simulink model "Proj3_P3"  (Simulink 8.6)
settings: Solver=ode45  StartTime=0.0  StopTime=90  FixedStep=1e-4  MaxStep=1e-4  RelTol=1e-3
values from neighbouring files (symbols this model uses):
  A = 3904    [main.m]
  ControlQs = 1    [main.m]
  ControlVwind = -1    [main.m]
  fl_rd_rated = L_m*I_sd_rated + L_r*I_rd_rated    [main.m]
  fl_rq_rated = L_m*I_sq_rated + L_r*I_rq_rated    [main.m]
  fl_sd_rated = L_s*I_sd_rated + L_m*I_rd_rated    [main.m]
  fl_sq_rated = L_s*I_sq_rated + L_m*I_rq_rated    [main.m]
  GearRatio = w_mech_rated / w_mech_opt    [main.m]
  J_turb = 2.4*10^6    (= 2400000)    [main.m]
  K_opt = Cp_opt * 0.5 * rho * A * R^3/lambda_opt^3    (= -inf)    [main.m]
  kii = w_c_i*sqrt(R_r^2+(sigma*L_r*w_c_i)^2)/sqrt(1+(kpi_by_kii*w_c_i)^2)    [main.m]
  kpi = kpi_by_kii * kii    [main.m]
  L_m = X_m /w_syn    (= 0.00228122085098)    [main.m]
  L_r = L_lr+L_m    (= 0.00240589222307)    [main.m]
  L_s = L_ls+L_m    (= 0.00241384997023)    [main.m]
  lambda_opt = lam    (= 0.01)    [main.m]
  p = 6    [main.m]
  Q_s_rated = (V_sd_rated)^2/(w_syn*L_s)+(L_m/L_s)*V_sd_rated*I_rq_rated    [main.m]
  R = 70.5/2    (= 35.25)    [main.m]
  R_r = 1.5e-3    (= 0.0015)    [main.m]
  R_s = 2e-3    (= 0.002)    [main.m]
  rho = 1.2    [main.m]
  sigma = 1-L_m^2/(L_s*L_r)    (= 0.10391703115)    [main.m]
  V_ll_rated = 690    [main.m]
  V_sd_prime_rated = V_rd_rated + s*w_syn*sigma*L_r*I_rq_rated    [main.m]
  V_sd_rated = V_ll_rated    (= 690)    [main.m]
  V_sq_prime_rated = V_rq_rated - s*w_syn*sigma*L_r*I_rd_rated    [main.m]
  v_wind = [12; 9; 6]    [main.m]
  w_mech_opt = lambda_opt*v_wind(1)/R    [main.m]
  w_mech_rated = (1-s)*w_syn/(p/2)    (= 124.407069082)    [main.m]
  w_syn = 2*pi*f_rated    (= 376.991118431)    [main.m]
settings Model: Creator=Admin  LastModifiedBy=XP
settings OptimizationCC: ExpressionDepthLimit=128
settings DebuggingCC: FcnCallInpInsideContextMsg=UseLocalSettings  StateNameClashWarn=none

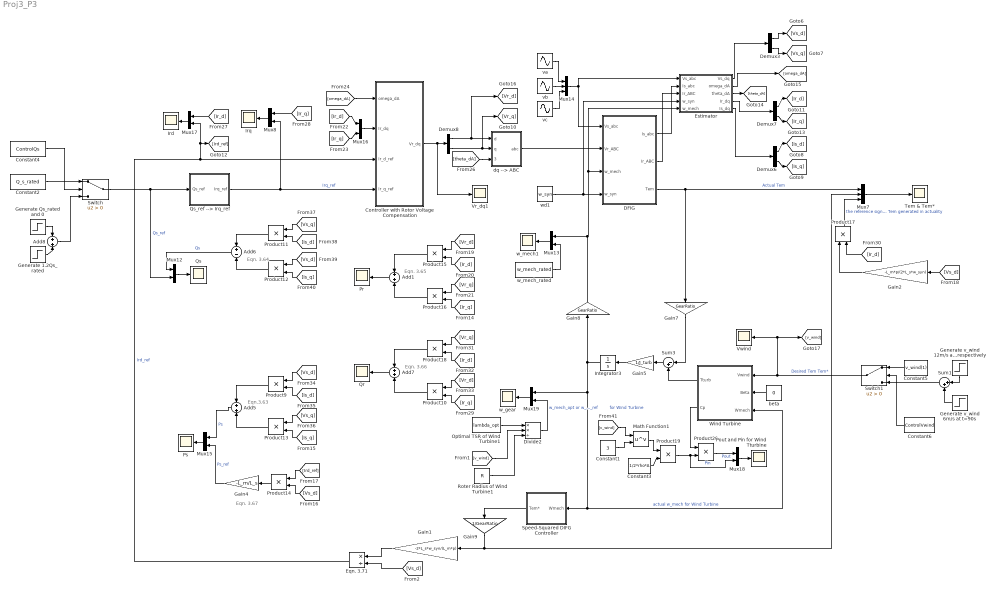
== system Proj3_P3 ==
  note: Eqn. 3.64
  note: Eqn. 3.66
  note: Eqn. 3.65
  note: Eqn.3.63
  note: Eqn. 3.67
  " Gain4" : Gain  Gain=-L_m/L_s
  " Gain5" : Gain  Gain=1/J_turb
  Add{1,5,7..8} (4 alike) : Sum
  Add6 : Sum  Inputs=+-
  Constant1 : Constant  Value=3
  Constant2 : Constant  Value=Q_s_rated
  Constant3 : Constant  Value=1/2*rho*A
  Constant4 : Constant  Value=ControlQs
  Constant5 : Constant  Value=v_wind(1)
  Constant6 : Constant  Value=ControlVwind
  Controller with Rotor Voltage Compensation : Subsystem
  DFIG : Subsystem
  Demux{3,6..8} (4 alike) : Demux  Outputs=2
  Divide2 : Product  Inputs=**/
  "Eqn. 3.71 " : Product  Inputs=*/
  Estimator : Subsystem
  Gain1 : Gain  Gain=-2*L_s*w_syn/(L_m*p)
  Gain2 : Gain  Gain=-L_m*p/(2*L_s*w_syn)
  Gain7 : Gain  Gain=GearRatio
  Gain8 : Gain  Gain=GearRatio
  Gain9 : Gain  Gain=1/GearRatio
  Generate Qs_rated and 0 : Step  Time=30  Before=Q_s_rated  After=0  SampleTime=0
  Generate 1.2Qs_rated : Step  Time=60  After=1.2*Q_s_rated  SampleTime=0
  Generate v_wind 12m/s and 9m/s at t=0s and t=60s respectively : Step  Time=30  Before=v_wind(1)  After=v_wind(2)  SampleTime=0
  Generate v_wind 6m/s at t=90s : Step  Time=60  After=v_wind(3)-v_wind(2)  SampleTime=0
  Integrator3 : Integrator  InitialCondition=w_mech_opt
  Ird : Scope
  Irq : Scope
  Math Function1 : Math  Operator=pow  SaturateOnIntegerOverflow=on
  Mux{8,12..13,15..19} (8 alike) : Mux  Inputs=2
  Mux14 : Mux  Inputs=3
  Mux7 : Mux  Inputs=3
  Optimal TSR of Wind Turbine1 : Constant  Value=lambda_opt
  Pout and Pin for Wind Tturbine : Scope
  Pr : Scope
  Product{9..20} (12 alike) : Product
  Ps : Scope
  Qr : Scope
  Qs : Scope
  Qs_ref --> Irq_ref : Subsystem
  Roter Radius of Wind Turbine1 : Constant  Value=R
  Speed-Squared DIFG Controller : Subsystem
  Sum1 : Sum  Inputs=|++
  Sum3 : Sum  Inputs=|-+
  Switch : Switch  Criteria=u2 > Threshold
  Switch1 : Switch  Criteria=u2 > Threshold
  Tem & Tem* : Scope
  Vr_dq1 : Scope
  Vwind : Scope
  Wind Turbine : Subsystem
  beta : Constant  Value=0
  dq --> ABC : Subsystem
  va : Sin  Amplitude=V_ll_rated*sqrt(2/3)  Frequency=2*pi*60  Phase=pi/2  SampleTime=0
  vb : Sin  Amplitude=V_ll_rated*sqrt(2/3)  Frequency=2*pi*60  Phase=pi/2-2*pi/3  SampleTime=0
  vc : Sin  Amplitude=V_ll_rated*sqrt(2/3)  Frequency=2*pi*60  Phase=pi/2+2*pi/3  SampleTime=0
  w_gear : Scope
  w_mech1 : Scope
  w_mech_rated : Constant  Value=w_mech_rated
  wd1 : Constant  Value=w_syn
  wires:
  dq --> ABC/1(abc) -> DFIG/2(Vr_ABC)
  vb/1 -> Mux14/2
  vc/1 -> Mux14/3
  va/1 -> Mux14/1
  Mux14/1 -> Estimator/1(Vs_abc), DFIG/1(Vs_abc)
  Demux8/1 -> dq --> ABC/1(d), [Vr_d]
  Demux8/2 -> [Vr_q], dq --> ABC/2(q)
  Controller with Rotor Voltage Compensation/1(Vr_dq) -> Vr_dq1/1, Demux8/1
  Mux17/1 -> Ird/1
  wd1/1 -> Estimator/4(w_syn), DFIG/4(w_syn)
  Estimator/1(Vs_dq) -> Demux3/1
  Mux7/1 -> Tem & Tem*/1
  "Eqn. 3.71 "/1 -> Controller with Rotor Voltage Compensation/3(Ir_d_ref), [Ird_ref], Mux17/2  "Ird_ref"
  Demux3/1 -> [Vs_d]
  Demux3/2 -> [Vs_q]
  Mux12/1 -> Qs/1
  DFIG/1(Is_abc) -> Estimator/2(Is_abc)
  DFIG/2(Ir_ABC) -> Estimator/3(Ir_ABC)
  Mux13/1 -> w_mech1/1
  w_mech_rated/1 -> Mux13/2
  Estimator/5(Is_dq) -> Demux6/1
  Demux6/1 -> [Is_d]
  Demux6/2 -> [Is_q]
  Add6/1 -> Mux12/1  "Qs"
  [Vs_q] -> Product11/1
  [Is_d] -> Product11/2
  [Vs_d] -> Product12/1
  [Is_q] -> Product12/2
  Product11/1 -> Add6/1
  Product12/1 -> Add6/2
  Switch/1 -> Mux12/2, Qs_ref --> Irq_ref/1(Qs_ref)  "Qs_ref"
  [Vs_d] -> Product9/1
  [Is_d] -> Product9/2
  [Vs_q] -> Product13/1
  [Is_q] -> Product13/2
  Product9/1 -> Add5/1
  Product13/1 -> Add5/2
  Add5/1 -> Mux15/1  "Ps"
  Estimator/2(omega_dA) -> [omega_dA]
  Gain8/1 -> Estimator/5(w_mech), DFIG/3(w_mech), Mux13/1
  [Vr_d] -> Product15/1
  [Ir_d] -> Product15/2
  [Vr_q] -> Product16/1
  [Ir_q] -> Product16/2
  Product15/1 -> Add1/1
  Product16/1 -> Add1/2
  Add1/1 -> Pr/1
  Estimator/4(Ir_dq) -> Demux7/1
  Demux7/1 -> [Ir_d]
  Demux7/2 -> [Ir_q]
  Estimator/3(theta_dA) -> [theta_dA]
  Mux16/1 -> Controller with Rotor Voltage Compensation/2(Ir_dq)
  [Ir_d] -> Mux16/1
  [Ir_q] -> Mux16/2
  [omega_dA] -> Controller with Rotor Voltage Compensation/1(omega_dA)
  [theta_dA] -> dq --> ABC/3(theta_dA)
  [Ir_d] -> Mux17/1
  Qs_ref --> Irq_ref/1(Irq_ref) -> Controller with Rotor Voltage Compensation/4(Ir_q_ref), Mux8/2  "Irq_ref"
  Mux8/1 -> Irq/1
  [Ir_q] -> Mux8/1
  [Vr_q] -> Product18/1
  [Ir_d] -> Product18/2
  [Vr_d] -> Product10/1
  [Ir_q] -> Product10/2
  Product18/1 -> Add7/1
  Product10/1 -> Add7/2
  Add7/1 -> Qr/1
  [Vs_d] -> Gain2/1
  [Ir_d] -> Product17/2
  Product17/1 -> Mux7/3  "the reference signal of Tem generated in actuality"
  Gain9/1 -> Gain1/1, Mux7/2  "Desired Tem Tem*"
  Gain2/1 -> Product17/1
  DFIG/3(Tem) -> Mux7/1, Gain7/1  "Actual Tem"
  Gain7/1 -> Sum3/1
  Sum3/1 -> " Gain5"/1
  " Gain5"/1 -> Integrator3/1
  Wind Turbine/1(Tturb) -> Sum3/2
  beta/1 -> Wind Turbine/2(Beta)
  [v_wind] -> Math Function1/1
  Constant1/1 -> Math Function1/2
  Constant3/1 -> Product19/2
  Math Function1/1 -> Product19/1
  Product19/1 -> Mux18/2, Product20/2  "Pin"
  Wind Turbine/2(Cp) -> Product20/1
  Product20/1 -> Mux18/1  "Pout"
  Mux18/1 -> Pout and Pin for Wind Tturbine/1
  Speed-Squared DIFG Controller/1(Tem*) -> Gain9/1
  Mux19/1 -> w_gear/1
  Divide2/1 -> Mux19/2  "w_mech_opt or w_mech_ref         for Wind Turbine"
  Integrator3/1 -> Gain8/1, Mux19/1, Speed-Squared DIFG Controller/1(Wmech), Wind Turbine/3(Wmech)  "actual w_mech for Wind Turbine"
  [v_wind] -> Divide2/2
  Optimal TSR of Wind Turbine1/1 -> Divide2/1
  Roter Radius of Wind Turbine1/1 -> Divide2/3
  Generate Qs_rated and 0/1 -> Add8/1
  Generate 1.2Qs_rated/1 -> Add8/2
  Constant2/1 -> Switch/1
  Add8/1 -> Switch/3
  Constant4/1 -> Switch/2
  Sum1/1 -> Switch1/3
  Generate v_wind 6m/s at t=90s/1 -> Sum1/2
  Generate v_wind 12m/s and 9m/s at t=0s and t=60s respectively/1 -> Sum1/1
  Constant5/1 -> Switch1/1
  [Vs_d] -> "Eqn. 3.71 "/2
  Gain1/1 -> "Eqn. 3.71 "/1
  Switch1/1 -> [v_wind], Vwind/1, Wind Turbine/1(Vwind)
  Constant6/1 -> Switch1/2
  [Vs_d] -> Product14/2
  [Ird_ref] -> Product14/1
  Product14/1 -> " Gain4"/1
  " Gain4"/1 -> Mux15/2  "Ps_ref"
  Mux15/1 -> Ps/1

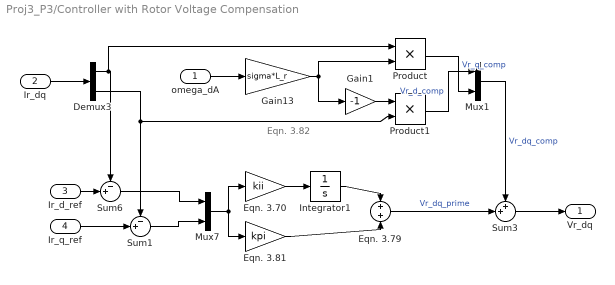
== system Proj3_P3/Controller with Rotor Voltage Compensation ==
  note: Eqn. 3.82
  omega_dA : Inport
  Ir_dq : Inport  Port=2
  Ir_d_ref : Inport  Port=3
  Ir_q_ref : Inport  Port=4
  "                       Eqn. 3.79" : Sum
  Demux3 : Demux  Outputs=2
  Eqn. 3.70 : Gain  Gain=kii
  Eqn. 3.81 : Gain  Gain=kpi
  Gain1 : Gain  Gain=-1
  Gain13 : Gain  Gain=sigma*L_r
  Integrator1 : Integrator  InitialCondition=[V_sd_prime_rated; V_sq_prime_rated]
  Mux1 : Mux  Inputs=2
  Mux7 : Mux  Inputs=2
  Product : Product
  Product1 : Product
  Sum1 : Sum  Inputs=-+|  SaturateOnIntegerOverflow=on  InputSameDT=on  OutDataTypeStr=Inherit: Same as first input
  Sum3 : Sum  Inputs=++|  SaturateOnIntegerOverflow=on  InputSameDT=on  OutDataTypeStr=Inherit: Same as first input
  Sum6 : Sum  Inputs=-+|  SaturateOnIntegerOverflow=on  InputSameDT=on  OutDataTypeStr=Inherit: Same as first input
  Vr_dq : Outport
  wires:
  Eqn. 3.70/1 -> Integrator1/1
  Integrator1/1 -> "                       Eqn. 3.79"/1
  Eqn. 3.81/1 -> "                       Eqn. 3.79"/2
  Mux7/1 -> Eqn. 3.81/1, Eqn. 3.70/1
  "                       Eqn. 3.79"/1 -> Sum3/2  "Vr_dq_prime"
  Demux3/2 -> Sum1/1, Product1/2
  Gain1/1 -> Product1/1
  Product1/1 -> Mux1/1  "Vr_d_comp"
  Gain13/1 -> Product/2, Gain1/1
  Product/1 -> Mux1/2  "Vr_q_comp"
  omega_dA/1 -> Gain13/1
  Ir_dq/1 -> Demux3/1
  Demux3/1 -> Sum6/1, Product/1
  Mux1/1 -> Sum3/1  "Vr_dq_comp"
  Sum3/1 -> Vr_dq/1
  Ir_d_ref/1 -> Sum6/2
  Ir_q_ref/1 -> Sum1/2
  Sum1/1 -> Mux7/2
  Sum6/1 -> Mux7/1

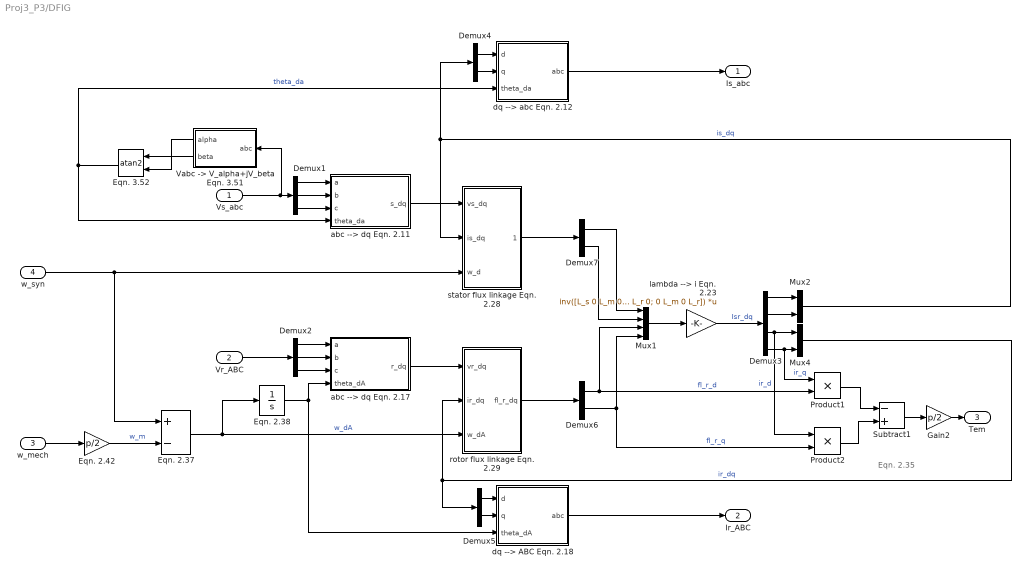
== system Proj3_P3/DFIG ==
  note: Eqn. 2.35
  Vs_abc : Inport
  Vr_ABC : Inport  Port=2
  w_mech : Inport  Port=3
  w_syn : Inport  Port=4
  Demux1 : Demux  Outputs=3
  Demux2 : Demux  Outputs=3
  Demux3 : Demux
  Demux{4..7} (4 alike) : Demux  Outputs=2
  Eqn. 2.37 : Sum  Inputs=+-
  Eqn. 2.38 : Integrator
  Eqn. 2.42 : Gain  Gain=p/2  SaturateOnIntegerOverflow=on  OutDataTypeStr=Inherit: Same as input  ParamDataTypeStr=Inherit: Same as input
  Eqn. 3.52 : Trigonometry  Operator=atan2
  Gain2 : Gain  Gain=p/2  SaturateOnIntegerOverflow=on  OutDataTypeStr=Inherit: Same as input  ParamDataTypeStr=Inherit: Same as input
  Mux1 : Mux
  Mux2 : Mux  Inputs=2
  Mux4 : Mux  Inputs=2
  Product1 : Product
  Product2 : Product
  Subtract1 : Sum  Inputs=-+
  "Vabc -> V_alpha+jV_beta Eqn. 3.51" : Subsystem
  abc --> dq Eqn. 2.11 : Subsystem
  abc --> dq Eqn. 2.17 : Subsystem
  dq --> ABC Eqn. 2.18 : Subsystem
  dq --> abc Eqn. 2.12 : Subsystem
  lambda --> i Eqn. 2.23 : Gain  Gain=inv([L_s 0 L_m 0; 0 L_s 0 L_m; L_m 0 L_r 0; 0 L_m 0 L_r])  Multiplication=Matrix(K*u)  SaturateOnIntegerOverflow=on  OutDataTypeStr=Inherit: Same as input  ParamDataTypeStr=Inherit: Same as input
  rotor flux linkage Eqn. 2.29 : Subsystem
  stator flux linkage Eqn. 2.28 : Subsystem
  Is_abc : Outport
  Ir_ABC : Outport  Port=2
  Tem : Outport  Port=3
  wires:
  Product2/1 -> Subtract1/2
  Vr_ABC/1 -> Demux2/1
  lambda --> i Eqn. 2.23/1 -> Demux3/1  "Isr_dq"
  Mux4/1 -> Demux5/1, rotor flux linkage Eqn. 2.29/2(ir_dq)  "ir_dq"
  Eqn. 2.37/1 -> rotor flux linkage Eqn. 2.29/3(w_dA), Eqn. 2.38/1  "w_dA"
  Demux4/1 -> dq --> abc Eqn. 2.12/1(d)
  Demux2/3 -> abc --> dq Eqn. 2.17/3(c)
  Demux2/1 -> abc --> dq Eqn. 2.17/1(a)
  Demux2/2 -> abc --> dq Eqn. 2.17/2(b)
  Eqn. 3.52/1 -> dq --> abc Eqn. 2.12/3(theta_da), abc --> dq Eqn. 2.11/4(theta_da)  "theta_da"
  Mux1/1 -> lambda --> i Eqn. 2.23/1
  Demux7/2 -> Mux1/2
  abc --> dq Eqn. 2.11/1(s_dq) -> stator flux linkage Eqn. 2.28/1(vs_dq)
  w_mech/1 -> Eqn. 2.42/1
  Demux4/2 -> dq --> abc Eqn. 2.12/2(q)
  Demux6/2 -> Mux1/4, Product2/2  "fl_r_q"
  Demux1/3 -> abc --> dq Eqn. 2.11/3(c)
  Eqn. 2.42/1 -> Eqn. 2.37/2  "w_m"
  Product1/1 -> Subtract1/1
  Eqn. 2.38/1 -> dq --> ABC Eqn. 2.18/3(theta_dA), abc --> dq Eqn. 2.17/4(theta_dA)
  Demux1/1 -> abc --> dq Eqn. 2.11/1(a)
  Demux5/1 -> dq --> ABC Eqn. 2.18/1(d)
  Demux5/2 -> dq --> ABC Eqn. 2.18/2(q)
  abc --> dq Eqn. 2.17/1(r_dq) -> rotor flux linkage Eqn. 2.29/1(vr_dq)
  rotor flux linkage Eqn. 2.29/1(fl_r_dq) -> Demux6/1
  Mux2/1 -> Demux4/1, stator flux linkage Eqn. 2.28/2(is_dq)  "is_dq"
  Demux6/1 -> Product1/2, Mux1/3  "fl_r_d"
  w_syn/1 -> stator flux linkage Eqn. 2.28/3(w_d), Eqn. 2.37/1
  dq --> abc Eqn. 2.12/1(abc) -> Is_abc/1
  Vs_abc/1 -> "Vabc -> V_alpha+jV_beta Eqn. 3.51"/1(abc), Demux1/1
  "Vabc -> V_alpha+jV_beta Eqn. 3.51"/2(beta) -> Eqn. 3.52/1
  dq --> ABC Eqn. 2.18/1(abc) -> Ir_ABC/1
  "Vabc -> V_alpha+jV_beta Eqn. 3.51"/1(alpha) -> Eqn. 3.52/2
  stator flux linkage Eqn. 2.28/1(fl_s_dq) -> Demux7/1
  Demux3/4 -> Product1/1, Mux4/2  "ir_q"
  Subtract1/1 -> Gain2/1
  Demux3/1 -> Mux2/1
  Demux3/3 -> Product2/1, Mux4/1  "ir_d"
  Demux3/2 -> Mux2/2
  Demux7/1 -> Mux1/1
  Gain2/1 -> Tem/1
  Demux1/2 -> abc --> dq Eqn. 2.11/2(b)

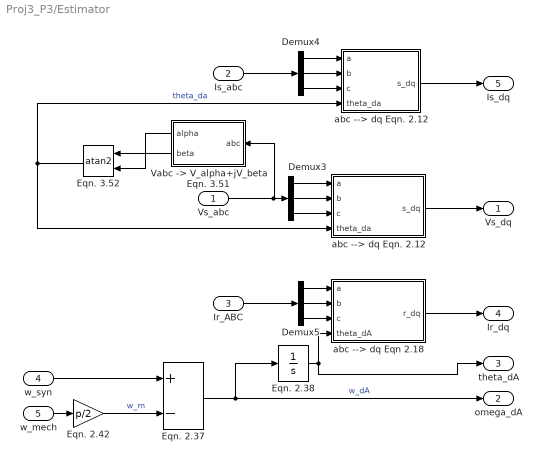
== system Proj3_P3/Estimator ==
  Vs_abc : Inport
  Is_abc : Inport  Port=2
  Ir_ABC : Inport  Port=3
  w_syn : Inport  Port=4
  w_mech : Inport  Port=5
  Demux3 : Demux  Outputs=3
  Demux4 : Demux  Outputs=3
  Demux5 : Demux  Outputs=3
  Eqn. 2.37 : Sum  Inputs=+-
  Eqn. 2.38 : Integrator
  Eqn. 2.42 : Gain  Gain=p/2  SaturateOnIntegerOverflow=on  OutDataTypeStr=Inherit: Same as input  ParamDataTypeStr=Inherit: Same as input
  Eqn. 3.52 : Trigonometry  Operator=atan2
  "Vabc -> V_alpha+jV_beta Eqn. 3.51" : Subsystem
  abc --> dq Eqn 2.18 : Subsystem
  abc --> dq Eqn. 2.12 : Subsystem
  "abc --> dq Eqn. 2.12 " : Subsystem
  Vs_dq : Outport
  omega_dA : Outport  Port=2
  theta_dA : Outport  Port=3
  Ir_dq : Outport  Port=4
  Is_dq : Outport  Port=5
  wires:
  Eqn. 3.52/1 -> "abc --> dq Eqn. 2.12 "/4(theta_da), abc --> dq Eqn. 2.12/4(theta_da)  "theta_da"
  "abc --> dq Eqn. 2.12 "/1(s_dq) -> Vs_dq/1
  Demux3/3 -> "abc --> dq Eqn. 2.12 "/3(c)
  Demux3/1 -> "abc --> dq Eqn. 2.12 "/1(a)
  Vs_abc/1 -> "Vabc -> V_alpha+jV_beta Eqn. 3.51"/1(abc), Demux3/1
  "Vabc -> V_alpha+jV_beta Eqn. 3.51"/2(beta) -> Eqn. 3.52/1
  "Vabc -> V_alpha+jV_beta Eqn. 3.51"/1(alpha) -> Eqn. 3.52/2
  Demux3/2 -> "abc --> dq Eqn. 2.12 "/2(b)
  Demux4/1 -> abc --> dq Eqn. 2.12/1(a)
  Demux4/2 -> abc --> dq Eqn. 2.12/2(b)
  Demux4/3 -> abc --> dq Eqn. 2.12/3(c)
  Is_abc/1 -> Demux4/1
  Demux5/1 -> abc --> dq Eqn 2.18/1(a)
  Demux5/2 -> abc --> dq Eqn 2.18/2(b)
  Demux5/3 -> abc --> dq Eqn 2.18/3(c)
  Ir_ABC/1 -> Demux5/1
  Eqn. 2.37/1 -> omega_dA/1, Eqn. 2.38/1  "w_dA"
  w_mech/1 -> Eqn. 2.42/1
  Eqn. 2.42/1 -> Eqn. 2.37/2  "w_m"
  w_syn/1 -> Eqn. 2.37/1
  Eqn. 2.38/1 -> theta_dA/1, abc --> dq Eqn 2.18/4(theta_dA)
  abc --> dq Eqn 2.18/1(r_dq) -> Ir_dq/1
  abc --> dq Eqn. 2.12/1(s_dq) -> Is_dq/1

== system Proj3_P3/Qs_ref --> Irq_ref ==
  note: Eqn. 3.72
  Qs_ref : Inport
  Constant1 : Constant  Value=V_sd_rated/(w_syn*L_m)
  Gain7 : Gain  Gain=L_s/(L_m*V_sd_rated)
  Sum2 : Sum  Inputs=|+-
  Irq_ref : Outport
  wires:
  Qs_ref/1 -> Gain7/1
  Constant1/1 -> Sum2/2
  Gain7/1 -> Sum2/1
  Sum2/1 -> Irq_ref/1  "Irq_ref"

== system Proj3_P3/Speed-Squared DIFG Controller ==
  Wmech : Inport
  "Tem*=Kopt * Wmech^2 Eqn. 4.91 " : Fcn  Expr=K_opt*u^2
  Tem* : Outport
  wires:
  "Tem*=Kopt * Wmech^2 Eqn. 4.91 "/1 -> Tem*/1
  Wmech/1 -> "Tem*=Kopt * Wmech^2 Eqn. 4.91 "/1

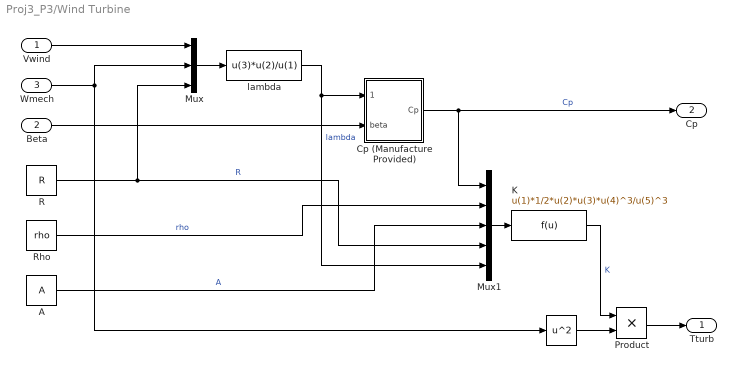
== system Proj3_P3/Wind Turbine ==
  Vwind : Inport
  Beta : Inport  Port=2
  Wmech : Inport  Port=3
  " " : Fcn  Expr=u^2
  A : Constant  Value=A
  Cp (Manufacture Provided) : Subsystem
  K : Fcn  Expr=u(1)*1/2*u(2)*u(3)*u(4)^3/u(5)^3
  Mux : Mux  Inputs=3
  Mux1 : Mux  Inputs=5
  Product : Product
  R : Constant  Value=R
  Rho : Constant  Value=rho
  lambda : Fcn  Expr=u(3)*u(2)/u(1)
  Tturb : Outport
  Cp : Outport  Port=2
  wires:
  lambda/1 -> Mux1/5, Cp (Manufacture Provided)/1(lambda)  "lambda"
  K/1 -> Product/1  "K"
  A/1 -> Mux1/3  "A"
  Mux1/1 -> K/1
  Mux/1 -> lambda/1
  Cp (Manufacture Provided)/1(Cp) -> Mux1/1, Cp/1  "Cp"
  " "/1 -> Product/2
  Product/1 -> Tturb/1
  Rho/1 -> Mux1/2  "rho"
  R/1 -> Mux/3, Mux1/4  "R"
  Vwind/1 -> Mux/1
  Wmech/1 -> Mux/2, " "/1
  Beta/1 -> Cp (Manufacture Provided)/2(beta)

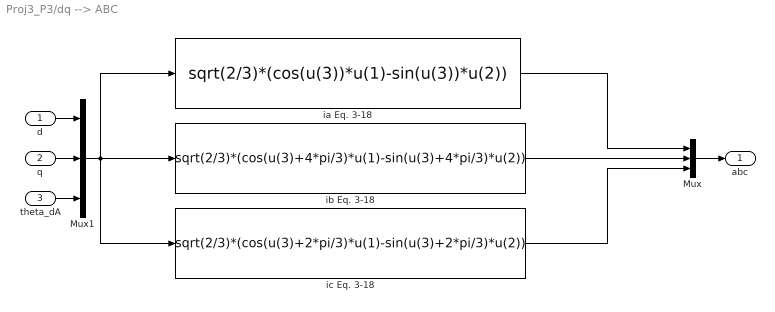
== system Proj3_P3/dq --> ABC ==
  d : Inport
  q : Inport  Port=2
  theta_dA : Inport  Port=3
  Mux : Mux  Inputs=3
  Mux1 : Mux  Inputs=3
  ia Eq. 3-18 : Fcn  Expr=sqrt(2/3)*(cos(u(3))*u(1)-sin(u(3))*u(2))
  ib Eq. 3-18 : Fcn  Expr=sqrt(2/3)*(cos(u(3)+4*pi/3)*u(1)-sin(u(3)+4*pi/3)*u(2))
  ic Eq. 3-18 : Fcn  Expr=sqrt(2/3)*(cos(u(3)+2*pi/3)*u(1)-sin(u(3)+2*pi/3)*u(2))
  abc : Outport
  wires:
  Mux/1 -> abc/1
  ia Eq. 3-18/1 -> Mux/1
  ic Eq. 3-18/1 -> Mux/3
  ib Eq. 3-18/1 -> Mux/2
  theta_dA/1 -> Mux1/3
  q/1 -> Mux1/2
  d/1 -> Mux1/1
  Mux1/1 -> ia Eq. 3-18/1, ib Eq. 3-18/1, ic Eq. 3-18/1

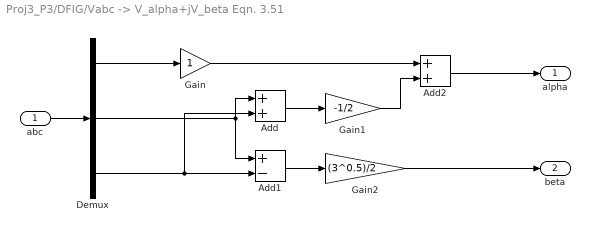
== system Proj3_P3/DFIG/Vabc -> V_alpha+jV_beta Eqn. 3.51 ==
  abc : Inport
  Add : Sum
  Add1 : Sum  Inputs=+-
  Add2 : Sum
  Demux : Demux  Outputs=3
  Gain : Gain
  Gain1 : Gain  Gain=-1/2
  Gain2 : Gain  Gain=(3^0.5)/2
  alpha : Outport
  beta : Outport  Port=2
  wires:
  Add/1 -> Gain1/1
  Add1/1 -> Gain2/1
  Demux/2 -> Add1/1, Add/1
  Demux/1 -> Gain/1
  Gain1/1 -> Add2/2
  Gain/1 -> Add2/1
  Add2/1 -> alpha/1
  Gain2/1 -> beta/1
  Demux/3 -> Add1/2, Add/2
  abc/1 -> Demux/1

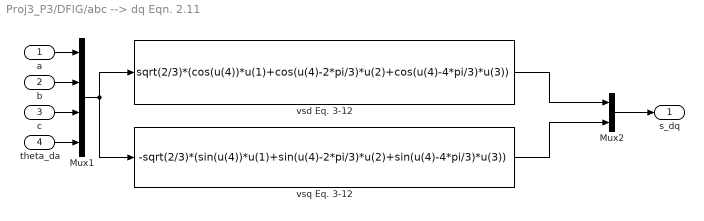
== system Proj3_P3/DFIG/abc --> dq Eqn. 2.11 ==
  a : Inport
  b : Inport  Port=2
  c : Inport  Port=3
  theta_da : Inport  Port=4
  Mux1 : Mux
  Mux2 : Mux  Inputs=2
  vsd Eq. 3-12 : Fcn  Expr=sqrt(2/3)*(cos(u(4))*u(1)+cos(u(4)-2*pi/3)*u(2)+cos(u(4)-4*pi/3)*u(3))
  vsq Eq. 3-12 : Fcn  Expr=-sqrt(2/3)*(sin(u(4))*u(1)+sin(u(4)-2*pi/3)*u(2)+sin(u(4)-4*pi/3)*u(3))
  s_dq : Outport
  wires:
  Mux1/1 -> vsd Eq. 3-12/1, vsq Eq. 3-12/1
  vsd Eq. 3-12/1 -> Mux2/1
  vsq Eq. 3-12/1 -> Mux2/2
  a/1 -> Mux1/1
  b/1 -> Mux1/2
  c/1 -> Mux1/3
  theta_da/1 -> Mux1/4
  Mux2/1 -> s_dq/1

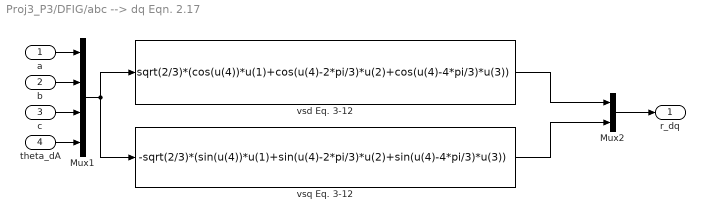
== system Proj3_P3/DFIG/abc --> dq Eqn. 2.17 ==
  a : Inport
  b : Inport  Port=2
  c : Inport  Port=3
  theta_dA : Inport  Port=4
  Mux1 : Mux
  Mux2 : Mux  Inputs=2
  vsd Eq. 3-12 : Fcn  Expr=sqrt(2/3)*(cos(u(4))*u(1)+cos(u(4)-2*pi/3)*u(2)+cos(u(4)-4*pi/3)*u(3))
  vsq Eq. 3-12 : Fcn  Expr=-sqrt(2/3)*(sin(u(4))*u(1)+sin(u(4)-2*pi/3)*u(2)+sin(u(4)-4*pi/3)*u(3))
  r_dq : Outport
  wires:
  Mux1/1 -> vsd Eq. 3-12/1, vsq Eq. 3-12/1
  vsd Eq. 3-12/1 -> Mux2/1
  vsq Eq. 3-12/1 -> Mux2/2
  a/1 -> Mux1/1
  b/1 -> Mux1/2
  c/1 -> Mux1/3
  theta_dA/1 -> Mux1/4
  Mux2/1 -> r_dq/1

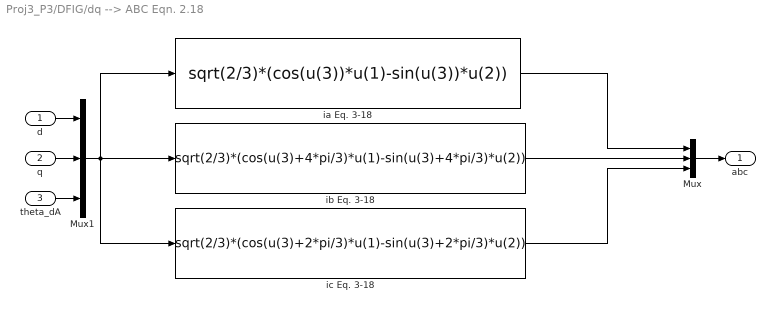
== system Proj3_P3/DFIG/dq --> ABC Eqn. 2.18 ==
  d : Inport
  q : Inport  Port=2
  theta_dA : Inport  Port=3
  Mux : Mux  Inputs=3
  Mux1 : Mux  Inputs=3
  ia Eq. 3-18 : Fcn  Expr=sqrt(2/3)*(cos(u(3))*u(1)-sin(u(3))*u(2))
  ib Eq. 3-18 : Fcn  Expr=sqrt(2/3)*(cos(u(3)+4*pi/3)*u(1)-sin(u(3)+4*pi/3)*u(2))
  ic Eq. 3-18 : Fcn  Expr=sqrt(2/3)*(cos(u(3)+2*pi/3)*u(1)-sin(u(3)+2*pi/3)*u(2))
  abc : Outport
  wires:
  Mux1/1 -> ic Eq. 3-18/1, ib Eq. 3-18/1, ia Eq. 3-18/1
  d/1 -> Mux1/1
  q/1 -> Mux1/2
  theta_dA/1 -> Mux1/3
  ib Eq. 3-18/1 -> Mux/2
  ic Eq. 3-18/1 -> Mux/3
  ia Eq. 3-18/1 -> Mux/1
  Mux/1 -> abc/1

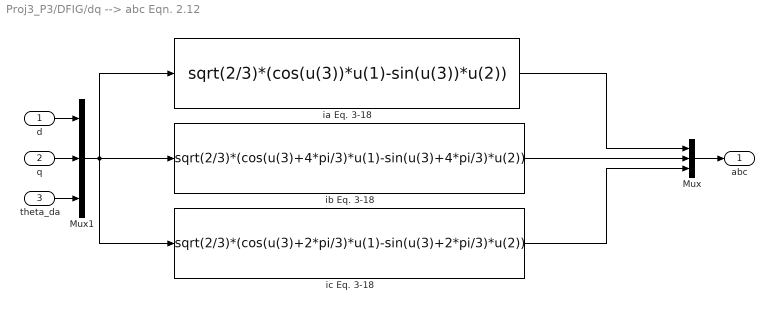
== system Proj3_P3/DFIG/dq --> abc Eqn. 2.12 ==
  d : Inport
  q : Inport  Port=2
  theta_da : Inport  Port=3
  Mux : Mux  Inputs=3
  Mux1 : Mux  Inputs=3
  ia Eq. 3-18 : Fcn  Expr=sqrt(2/3)*(cos(u(3))*u(1)-sin(u(3))*u(2))
  ib Eq. 3-18 : Fcn  Expr=sqrt(2/3)*(cos(u(3)+4*pi/3)*u(1)-sin(u(3)+4*pi/3)*u(2))
  ic Eq. 3-18 : Fcn  Expr=sqrt(2/3)*(cos(u(3)+2*pi/3)*u(1)-sin(u(3)+2*pi/3)*u(2))
  abc : Outport
  wires:
  Mux1/1 -> ic Eq. 3-18/1, ib Eq. 3-18/1, ia Eq. 3-18/1
  d/1 -> Mux1/1
  q/1 -> Mux1/2
  theta_da/1 -> Mux1/3
  ib Eq. 3-18/1 -> Mux/2
  ic Eq. 3-18/1 -> Mux/3
  ia Eq. 3-18/1 -> Mux/1
  Mux/1 -> abc/1

== system Proj3_P3/DFIG/rotor flux linkage Eqn. 2.29 ==
  note: Eq. 3-39
      | Fig. 3-7
  vr_dq : Inport
  ir_dq : Inport  Port=2
  w_dA : Inport  Port=3
  Gain : Gain  Gain=R_r  SaturateOnIntegerOverflow=on  OutDataTypeStr=Inherit: Same as input  ParamDataTypeStr=Inherit: Same as input
  Integrator1 : Integrator  InitialCondition=[fl_rd_rated;fl_rq_rated]
  Product : Product  SaturateOnIntegerOverflow=on  RndMeth=Zero  InputSameDT=on  OutDataTypeStr=Inherit: Same as first input
  Sum : Sum  Inputs=-+-  SaturateOnIntegerOverflow=on  InputSameDT=on  OutDataTypeStr=Inherit: Same as first input
  "[Mrotate] [0 -1  1 0] Eq. 3-37" : Gain  Gain=[0 -1; 1 0]  Multiplication=Matrix(K*u)  SaturateOnIntegerOverflow=on  OutDataTypeStr=Inherit: Same as input  ParamDataTypeStr=Inherit: Same as input
  fl_r_dq : Outport
  wires:
  Gain/1 -> Sum/3
  ir_dq/1 -> Gain/1
  vr_dq/1 -> Sum/2
  w_dA/1 -> Product/1
  Product/1 -> Sum/1
  "[Mrotate] [0 -1  1 0] Eq. 3-37"/1 -> Product/2
  Integrator1/1 -> fl_r_dq/1, "[Mrotate] [0 -1  1 0] Eq. 3-37"/1  "fl_r_dq"
  Sum/1 -> Integrator1/1

== system Proj3_P3/DFIG/stator flux linkage Eqn. 2.28 ==
  note: Eq. 3-38
      | Fig. 3-7
  vs_dq : Inport
  is_dq : Inport  Port=2
  w_d : Inport  Port=3
  Gain : Gain  Gain=R_s  SaturateOnIntegerOverflow=on  OutDataTypeStr=Inherit: Same as input  ParamDataTypeStr=Inherit: Same as input
  Integrator1 : Integrator  InitialCondition=[fl_sd_rated; fl_sq_rated]
  Product : Product  SaturateOnIntegerOverflow=on  RndMeth=Zero  InputSameDT=on  OutDataTypeStr=Inherit: Same as first input
  Sum : Sum  Inputs=-+-  SaturateOnIntegerOverflow=on  InputSameDT=on  OutDataTypeStr=Inherit: Same as first input
  "[Mrotate] [0 -1  1 0] Eq. 3-36 " : Gain  Gain=[0 -1; 1 0]  Multiplication=Matrix(K*u)  SaturateOnIntegerOverflow=on  OutDataTypeStr=Inherit: Same as input  ParamDataTypeStr=Inherit: Same as input
  fl_s_dq : Outport
  wires:
  Sum/1 -> Integrator1/1
  Integrator1/1 -> "[Mrotate] [0 -1  1 0] Eq. 3-36 "/1, fl_s_dq/1  "fl_s_dq"
  "[Mrotate] [0 -1  1 0] Eq. 3-36 "/1 -> Product/2
  Product/1 -> Sum/1
  w_d/1 -> Product/1
  vs_dq/1 -> Sum/2
  is_dq/1 -> Gain/1
  Gain/1 -> Sum/3

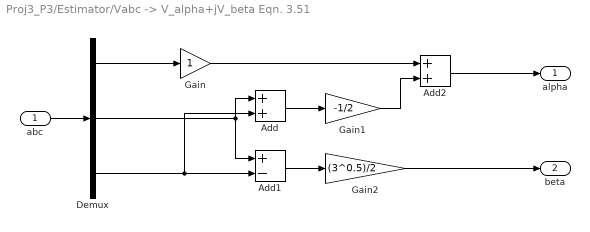
== system Proj3_P3/Estimator/Vabc -> V_alpha+jV_beta Eqn. 3.51 ==
  abc : Inport
  Add : Sum
  Add1 : Sum  Inputs=+-
  Add2 : Sum
  Demux : Demux  Outputs=3
  Gain : Gain
  Gain1 : Gain  Gain=-1/2
  Gain2 : Gain  Gain=(3^0.5)/2
  alpha : Outport
  beta : Outport  Port=2
  wires:
  Add/1 -> Gain1/1
  Add1/1 -> Gain2/1
  Demux/2 -> Add1/1, Add/1
  Demux/1 -> Gain/1
  Gain1/1 -> Add2/2
  Gain/1 -> Add2/1
  Add2/1 -> alpha/1
  Gain2/1 -> beta/1
  Demux/3 -> Add1/2, Add/2
  abc/1 -> Demux/1

== system Proj3_P3/Estimator/abc --> dq Eqn 2.18 ==
  a : Inport
  b : Inport  Port=2
  c : Inport  Port=3
  theta_dA : Inport  Port=4
  Mux1 : Mux
  Mux2 : Mux  Inputs=2
  vsd Eq. 3-12 : Fcn  Expr=sqrt(2/3)*(cos(u(4))*u(1)+cos(u(4)-2*pi/3)*u(2)+cos(u(4)-4*pi/3)*u(3))
  vsq Eq. 3-12 : Fcn  Expr=-sqrt(2/3)*(sin(u(4))*u(1)+sin(u(4)-2*pi/3)*u(2)+sin(u(4)-4*pi/3)*u(3))
  r_dq : Outport
  wires:
  Mux1/1 -> vsd Eq. 3-12/1, vsq Eq. 3-12/1
  vsd Eq. 3-12/1 -> Mux2/1
  vsq Eq. 3-12/1 -> Mux2/2
  a/1 -> Mux1/1
  b/1 -> Mux1/2
  c/1 -> Mux1/3
  theta_dA/1 -> Mux1/4
  Mux2/1 -> r_dq/1

== system Proj3_P3/Estimator/abc --> dq Eqn. 2.12 ==
  a : Inport
  b : Inport  Port=2
  c : Inport  Port=3
  theta_da : Inport  Port=4
  Mux1 : Mux
  Mux2 : Mux  Inputs=2
  vsd Eq. 3-12 : Fcn  Expr=sqrt(2/3)*(cos(u(4))*u(1)+cos(u(4)-2*pi/3)*u(2)+cos(u(4)-4*pi/3)*u(3))
  vsq Eq. 3-12 : Fcn  Expr=-sqrt(2/3)*(sin(u(4))*u(1)+sin(u(4)-2*pi/3)*u(2)+sin(u(4)-4*pi/3)*u(3))
  s_dq : Outport
  wires:
  Mux1/1 -> vsd Eq. 3-12/1, vsq Eq. 3-12/1
  vsd Eq. 3-12/1 -> Mux2/1
  vsq Eq. 3-12/1 -> Mux2/2
  a/1 -> Mux1/1
  b/1 -> Mux1/2
  c/1 -> Mux1/3
  theta_da/1 -> Mux1/4
  Mux2/1 -> s_dq/1

== system Proj3_P3/Estimator/abc --> dq Eqn. 2.12  ==
  a : Inport
  b : Inport  Port=2
  c : Inport  Port=3
  theta_da : Inport  Port=4
  Mux1 : Mux
  Mux2 : Mux  Inputs=2
  vsd Eq. 3-12 : Fcn  Expr=sqrt(2/3)*(cos(u(4))*u(1)+cos(u(4)-2*pi/3)*u(2)+cos(u(4)-4*pi/3)*u(3))
  vsq Eq. 3-12 : Fcn  Expr=-sqrt(2/3)*(sin(u(4))*u(1)+sin(u(4)-2*pi/3)*u(2)+sin(u(4)-4*pi/3)*u(3))
  s_dq : Outport
  wires:
  Mux1/1 -> vsd Eq. 3-12/1, vsq Eq. 3-12/1
  vsd Eq. 3-12/1 -> Mux2/1
  vsq Eq. 3-12/1 -> Mux2/2
  a/1 -> Mux1/1
  b/1 -> Mux1/2
  c/1 -> Mux1/3
  theta_da/1 -> Mux1/4
  Mux2/1 -> s_dq/1

== system Proj3_P3/Wind Turbine/Cp (Manufacture Provided) ==
  note: % Cp Model Terms
      | c1=0.52;
      | c2=116;
      | c3=0.4;
      | c4=5;
      | c5=21;
      | c6=0.0068;
  lambda : Inport
  beta : Inport  Port=2
  Fcn2 : Fcn  Expr=1/(1/(u(1)+0.08*u(2))-0.035/(u(2)^3+1))
  Fcn3 : Fcn  Expr=0.52*(116/u(2)-0.4*u(3)-5)*exp(-21/u(2))+0.0068*u(1)
  Mux2 : Mux  Inputs=2
  Mux3 : Mux  Inputs=3
  Cp : Outport
  wires:
  Fcn3/1 -> Cp/1
  Mux2/1 -> Fcn2/1
  beta/1 -> Mux2/2, Mux3/3
  Mux3/1 -> Fcn3/1
  lambda/1 -> Mux3/1, Mux2/1
  Fcn2/1 -> Mux3/2  "lambda_i"
